simulink model "FSF"  (R2020b)
settings: Solver=VariableStepAuto  StartTime=0.0  StopTime=tstop  RelTol=1e-9
undefined symbols (not defined in the file): A, B, input_select, K, t_end, Wc_sim, x0
libraries: simulink x1
settings Model: Creator=domin  LastModifiedBy=domin

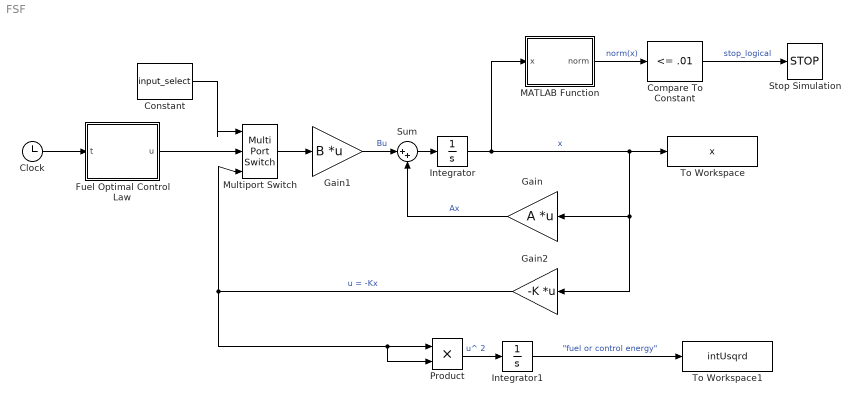
== system FSF ==
  Clock : Clock
  Compare To Constant : simulink/Logic and Bit Operations/Compare To Constant  relop=<=  const=.01  OutDataTypeStr=boolean
  Constant : Constant  Value=input_select
  Fuel Optimal Control Law : MATLAB Function  TreatAsAtomicUnit=on
  Gain : Gain  Gain=A  Multiplication=Matrix(K*u)
  Gain1 : Gain  Gain=B  Multiplication=Matrix(K*u)
  Gain2 : Gain  Gain=-K  Multiplication=Matrix(K*u)
  Integrator : Integrator  InitialCondition=x0
  Integrator1 : Integrator
  MATLAB Function : MATLAB Function  TreatAsAtomicUnit=on
  Multiport Switch : MultiPortSwitch  Inputs=2
  Product : Product
  Stop Simulation : Stop
  Sum : Sum  Inputs=|++
  To Workspace : ToWorkspace  VariableName=x  SampleTime=-1
  To Workspace1 : ToWorkspace  VariableName=intUsqrd  SampleTime=-1
  wires:
  Gain/1 -> Sum/2  "Ax"
  Gain1/1 -> Sum/1  "Bu"
  Integrator/1 -> MATLAB Function/1(x), To Workspace/1, Gain2/1, Gain/1  "x"
  Gain2/1 -> Multiport Switch/3, Product/1, Product/2  "u = -Kx"
  Sum/1 -> Integrator/1
  Product/1 -> Integrator1/1  "u^ 2"
  Integrator1/1 -> To Workspace1/1  "\"fuel or control energy\""
  MATLAB Function/1(norm) -> Compare To Constant/1  "norm(x)"
  Compare To Constant/1 -> Stop Simulation/1  "stop_logical"
  Constant/1 -> Multiport Switch/1
  Multiport Switch/1 -> Gain1/1
  Fuel Optimal Control Law/1(u) -> Multiport Switch/2
  Clock/1 -> Fuel Optimal Control Law/1(t)

== matlab function FSF/Fuel Optimal Control Law ==
  data: t input; u output; A parameter; B parameter; x0 parameter; t_end parameter; Wc_sim parameter
function u = fuel_opt(t,A,B,x0,t_end, Wc_sim)

    u = -(B')*expm(A'*(t_end-t))*(Wc_sim\expm(A*t_end)*x0);

== matlab function FSF/MATLAB Function ==
  data: x input; norm output
function norm = norm(x)

x = [x(1);x(2);x(3);x(4)];
norm = sqrt(x'*x);
